simulink model "ACC_System"  (R2022b)
settings: configuration reference "ACC_AutosarConfig" (kept outside this file)
model workspace (MATLAB code in the model file):
  | cmdLim = Simulink.Parameter;
  | cmdLim.Value = 15;
  | cmdLim.Description = 'Limit for controlling the maximum surface command angle.';
  | cmdLim.Min = 0;
  | cmdLim.Max = 90;
  | cmdLim.DocUnits = 'deg';
  | 
  | dispGain = Simulink.Parameter;
  | dispGain.Value = 0.75;
  | dispGain.Description = 'Gain applied to the displacement error.';
  | dispGain.Min = 0;
  | dispGain.Max = [];
  | dispGain.DocUnits = 'deg/sec/deg';
  | 
  | dispLim = Simulink.Parameter;
  | dispLim.Value = 30;
  | dispLim.Description = 'Limit for controlling the maximum commanded angle.';
  | dispLim.Min = 0;
  | dispLim.Max = 180;
  | dispLim.DocUnits = 'deg';
  | 
  | intGain = Simulink.Parameter;
  | intGain.Value = 0.5;
  | intGain.Description = 'Gain applied to the integral error.';
  | intGain.Min = 0;
  | intGain.Max = [];
  | intGain.DocUnits = 'deg/sec/deg/sec';
  | 
  | intLim = Simulink.Parameter;
  | intLim.Value = 5;
  | intLim.Description = 'Limit for controlling the maximum commanded angle.';
  | intLim.Min = 0;
  | intLim.Max = 90;
  | intLim.DocUnits = 'deg';
  | 
  | rateGain = Simulink.Parameter;
  | rateGain.Value = 2;
  | rateGain.Description = 'Gain applied to the rate error.';
  | rateGain.Min = 0;
  | rateGain.Max = [];
  | rateGain.DocUnits = 'deg/deg/sec';
  | 
  | rateLim = Simulink.Parameter;
  | rateLim.Value = 6;
  | rateLim.Description = 'Limit for controlling the maximum commanded angle.';
  | rateLim.Min = 0;
  | rateLim.Max = 180;
  | rateLim.DocUnits = 'deg/sec';
  | 
  | hdgGain = Simulink.Parameter;
  | hdgGain.Value = 0.015;
libraries: autosarlibdem x1, autosarlibnvm x1
settings Model: RequirementInfo={} %GIDa_fe9045fd_0412_4b6e_8206_617cc20e6fde  DataDictionary=ACC_DD.sldd  FPTRunName=Active  Creator=MAAM  LastModifiedBy=MAAM
settings ConfigSetRef: SourceName=ACC_AutosarConfig

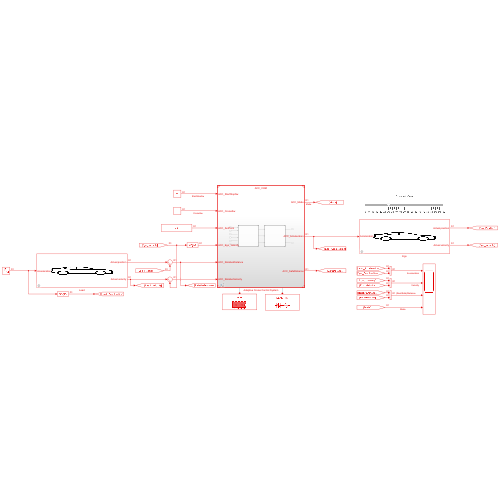
[thumbnail: Simulink's stored preview of the top-level diagram]
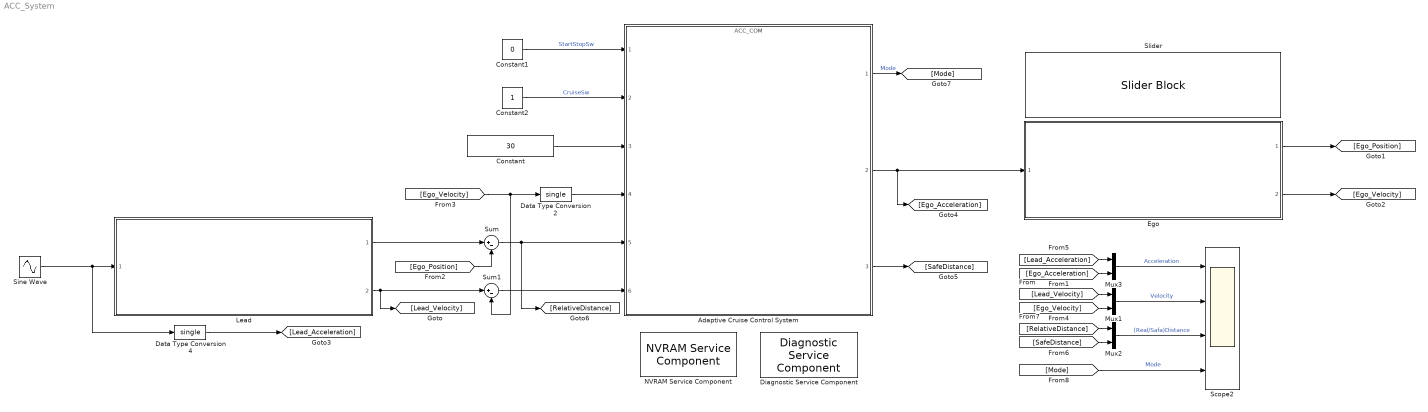
== system ACC_System ==
  Adaptive Cruise Control System : ModelReference  ModelNameDialog=ACC_COM.slx  SimulationMode=Normal  ModelReferenceVersion=1.11
  Constant : Constant  Value=30  OutDataTypeStr=single  SampleTime=-1
  Constant1 : Constant  Value=0  OutDataTypeStr=boolean  SampleTime=-1
  Constant2 : Constant  OutDataTypeStr=boolean  SampleTime=-1
  Data Type Conversion2 : DataTypeConversion  OutDataTypeStr=single  SaturateOnIntegerOverflow=off  RndMeth=Floor
  Data Type Conversion4 : DataTypeConversion  OutDataTypeStr=single  SaturateOnIntegerOverflow=off  RndMeth=Floor
  Diagnostic Service Component : autosarlibdem/Diagnostic Service Component  ClientPortNames={'ACC_Fail'}  ClientPortPortDefinedArguments={'1'}  MaxEventId=5  MaxFID=1  DemDebounceCounterIncrementStepSize=1  DemDebounceCounterDecrementStepSize=1  DemDebounceCounterFailedThreshold=2  DemDebounceCounterPassedThreshold=-1  InhibitionMatrix=[0 0 0 0 0 0 0 0 0 0 0;0 0 0 0 0 0 0 0 0 0 0;0 0 0 0 0 0 0 0 0 0 0;0 0 0 0 0 0 0 0 0 0 0;0 0 0 0 0 0 0 0 0 0 0;0 0 0 0 0 0 0 0 0 0 0;0 0 0 0 0 0 0 0 0 0 0;0 0 0 0 0 0 0 0 0 0 0;0 0 0 0 0 0 0 0 0 0 0;0 0 0 0 0 0 0 0 0 0 0;0 0 0 0 0 0 0 0 0 0 0]  EnableConditionIndexes=zeros(257,'uint8')  StorageConditionIndexes=zeros(257,'uint8')
  Ego : Subsystem  ReferencedSubsystem=Car  InitPos=10  InitVol=20
  Lead : Subsystem  ReferencedSubsystem=Car  InitPos=50  InitVol=25
  Mux1 : Mux  Inputs=2
  Mux2 : Mux  Inputs=2
  Mux3 : Mux  Inputs=2
  NVRAM Service Component : autosarlibnvm/NVRAM Service Component  ClientPortNames={'ACC_DefaultDistance_NvMService', 'ACC_TimeGap_NvMService', 'ACC_threshold_ID_NvMService'}  ClientPortPortDefinedArguments={'126', '225', '125'}  MaxBlockId=10  NvInitValues={'0', '0', '0', '0', '0', '0', '0', '0', '0', '0', '0', '0', '0', '0', '0', '0', '0', '0', '0', '0', '0', '0', '0', '0', '0', '0', '0', '0', '0', '0', '0', '0', '0', '0', '0', '0', '0', '0', '0', '0', '0', '0', '0', '0', '0', '0', '0', '0', '0', '0', '0', '0', '0', '0', '0', '0', '0', '0', '0', '0', '0', '0', '0', '0', '0', '0', '0', '0', '0', '0', '0', '0', '0', '0', '0', '0', '0', '0', '0', '0', '0', '0', '0', '0', '0', '0', '0', '0', '0', '0', '0', '0', '0', '0', '0', '0', '0', '0', '0', '0', '0', '0', '0', '0', '0', '0', '0', '0', '0', '0', '0', '0', '0', '0', '0', '0', '0', '0', '0', '0', '0', '0', '0', '0', '1', '10', '0', '0', '0', '0', '0', '0', '0', '0', '0', '0', '0', '0', '0', '0', '0', '0', '0', '0', '0', '0', '0', '0', '0', '0', '0', '0', '0', '0', '0', '0', '0', '0', '0', '0', '0', '0', '0', '0', '0', '0', '0', '0', '0', '0', '0', '0', '0', '0', '0', '0', '0', '0', '0', '0', '0', '0', '0', '0', '0', '0', '0', '0', '0', '0', '0', '0', '0', '0', '0', '0', '0', '0', '0', '0', '0', '0', '0', '0', '0', '0', '0', '0', '0', '0', '0', '0', '0', '0', '0', '0', '0', '0', '0', '0', '0', '0', '0', '0', '14'}
  Scope2 : Scope  NumInputPorts=4
  Sine Wave : Sin  Amplitude=4
  Slider : SliderBlock
  Sum : Sum  Inputs=|+-  OutDataTypeStr=single
  Sum1 : Sum  Inputs=|+-  OutDataTypeStr=single
  wires:
  Adaptive Cruise Control System/2 -> Ego/1, [Ego_Acceleration]
  Sum/1 -> Adaptive Cruise Control System/5, [RelativeDistance]
  Mux2/1 -> Scope2/3  "(Real/Safa)Distance"
  Mux1/1 -> Scope2/2  "Velocity"
  Mux3/1 -> Scope2/1  "Acceleration"
  Ego/1 -> [Ego_Position]
  Lead/1 -> Sum/1
  Lead/2 -> Sum1/1, [Lead_Velocity]
  Ego/2 -> [Ego_Velocity]
  Constant/1 -> Adaptive Cruise Control System/3
  Data Type Conversion2/1 -> Adaptive Cruise Control System/4
  Sum1/1 -> Adaptive Cruise Control System/6
  Adaptive Cruise Control System/3 -> [SafeDistance]
  Adaptive Cruise Control System/1 -> [Mode]  "Mode"
  Constant1/1 -> Adaptive Cruise Control System/1  "StartStopSw"
  Constant2/1 -> Adaptive Cruise Control System/2  "CruiseSw"
  [Lead_Velocity] -> Mux1/1
  [Ego_Position] -> Sum/2
  [Ego_Velocity] -> Data Type Conversion2/1, Sum1/2
  [Ego_Velocity] -> Mux1/2
  [Ego_Acceleration] -> Mux3/2
  [Lead_Acceleration] -> Mux3/1
  [SafeDistance] -> Mux2/2
  [RelativeDistance] -> Mux2/1
  [Mode] -> Scope2/4  "Mode"
  Data Type Conversion4/1 -> [Lead_Acceleration]
  Sine Wave/1 -> Lead/1, Data Type Conversion4/1
